simulink model "SYSTEMS"  (R2024b)
settings: configuration reference "STM32H7_Config" (kept outside this file)
settings Model: DataDictionary=Master_Dictionary.sldd  EnableAccessToBaseWorkspace=off  Creator=torni  LastModifiedBy=oxbro
settings ConfigSetRef: SourceName=STM32H7_Config

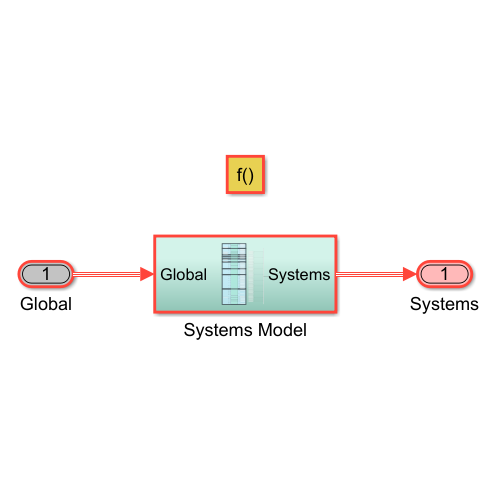
[thumbnail: Simulink's stored preview of the top-level diagram]
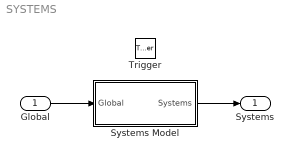
== system SYSTEMS ==
  "Global " : Inport  OutDataTypeStr=Bus: Global
  Trigger : TriggerPort  TriggerType=function-call  VariantControl=Variant  PortDimensions=1  TriggerSignalSampleTime=[0.003333333333333334,0]  OutDataTypeStr=double
  Systems Model : Subsystem
  Systems : Outport  OutDataTypeStr=Bus: SystemsBus  VectorParamsAs1DForOutWhenUnconnected=off
  wires:
  "Global "/1 -> Systems Model/1(Global)
  Systems Model/1(Systems) -> Systems/1

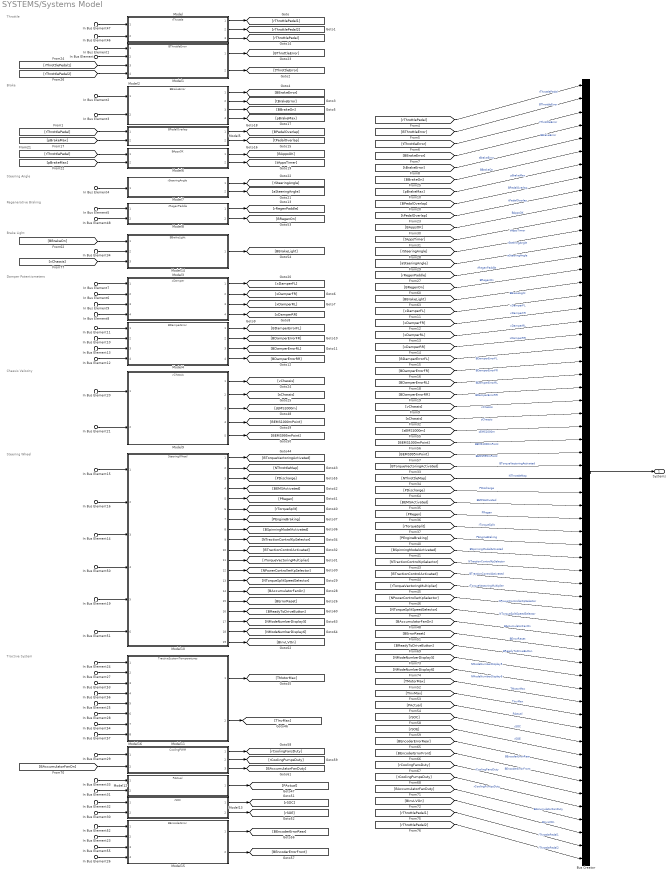
== system SYSTEMS/Systems Model ==
  note: Chassis Velocity
  note: Damper Potentiometers
  note: Regenerative Braking
  note: Steering Wheel
  note: Steering Angle
  note: Brake
  note: Throttle
  note: Tractive System
  note: Brake Light
  In Bus Element46 : Inport  PortName=Global  Element=SensorSignalsBus.VThrottlePedal2
  In Bus Element : Inport  PortName=Global  Element=SensorSignalsBus.VThrottlePedal2
  In Bus Element47 : Inport  PortName=Global  Element=SensorSignalsBus.VThrottlePedal1
  In Bus Element1 : Inport  PortName=Global  Element=SensorSignalsBus.VThrottlePedal1
  In Bus Element2 : Inport  PortName=Global  Element=SensorSignalsBus.pBrakeF
  In Bus Element3 : Inport  PortName=Global  Element=SensorSignalsBus.pBrakeR
  In Bus Element4 : Inport  PortName=Global  Element=SensorSignalsBus.VSteeringAngle
  In Bus Element5 : Inport  PortName=Global  Element=SensorSignalsBus.VRegenPaddle1
  In Bus Element48 : Inport  PortName=Global  Element=SensorSignalsBus.VRegenPaddle2
  In Bus Element6 : Inport  PortName=Global  Element=SensorSignalsBus.VDamperPotentiometerFR
  In Bus Element10 : Inport  PortName=Global  Element=SensorSignalsBus.VDamperPotentiometerFR
  In Bus Element7 : Inport  PortName=Global  Element=SensorSignalsBus.VDamperPotentiometerFL
  In Bus Element11 : Inport  PortName=Global  Element=SensorSignalsBus.VDamperPotentiometerFL
  In Bus Element8 : Inport  PortName=Global  Element=SensorSignalsBus.VDamperPotentiometerRR
  In Bus Element12 : Inport  PortName=Global  Element=SensorSignalsBus.VDamperPotentiometerRR
  In Bus Element9 : Inport  PortName=Global  Element=SensorSignalsBus.VDamperPotentiometerRL
  In Bus Element13 : Inport  PortName=Global  Element=SensorSignalsBus.VDamperPotentiometerRL
  In Bus Element16 : Inport  PortName=Global  Element=SensorSignalsBus.NDisplayNumberDDU7
  In Bus Element19 : Inport  PortName=Global  Element=SensorSignalsBus.BSteeringWheelButton4
  In Bus Element50 : Inport  PortName=Global  Element=SensorSignalsBus.BSteeringWheelButton5
  In Bus Element51 : Inport  PortName=Global  Element=SensorSignalsBus.BSteeringWheelButton6
  In Bus Element14 : Inport  PortName=Global  Element=SensorSignalsBus.BSteeringWheelButton2
  In Bus Element15 : Inport  PortName=Global  Element=SensorSignalsBus.BSteeringWheelButton7
  In Bus Element20 : Inport  PortName=Global  Element=WheelSpeedsBus.vWheelRL
  In Bus Element21 : Inport  PortName=Global  Element=WheelSpeedsBus.vWheelRR
  In Bus Element23 : Inport  PortName=Global  Element=InverterSignalsBus.InverterFLSignalsBus.NInvDTCFL
  In Bus Element24 : Inport  PortName=Global  Element=InverterSignalsBus.InverterFLSignalsBus.TMotorFL
  In Bus Element25 : Inport  PortName=Global  Element=InverterSignalsBus.InverterFLSignalsBus.TInvFL
  In Bus Element26 : Inport  PortName=Global  Element=InverterSignalsBus.InverterFRSignalsBus.NInvDTCFR
  In Bus Element27 : Inport  PortName=Global  Element=InverterSignalsBus.InverterFRSignalsBus.TMotorFR
  In Bus Element28 : Inport  PortName=Global  Element=InverterSignalsBus.InverterFRSignalsBus.TInvFR
  In Bus Element52 : Inport  PortName=Global  Element=InverterSignalsBus.InverterRLSignalsBus.NInvDTCRL
  In Bus Element53 : Inport  PortName=Global  Element=InverterSignalsBus.InverterRLSignalsBus.TMotorRL
  In Bus Element54 : Inport  PortName=Global  Element=InverterSignalsBus.InverterRLSignalsBus.TInvRL
  In Bus Element33 : Inport  PortName=Global  Element=InverterSignalsBus.InverterRLSignalsBus.VDCInvRL
  In Bus Element55 : Inport  PortName=Global  Element=InverterSignalsBus.InverterRRSignalsBus.NInvDTCRR
  In Bus Element56 : Inport  PortName=Global  Element=InverterSignalsBus.InverterRRSignalsBus.TMotorRR
  In Bus Element57 : Inport  PortName=Global  Element=InverterSignalsBus.InverterRRSignalsBus.TInvRR
  In Bus Element29 : Inport  PortName=Global  Element=BMSSignalsBus.TCellMax
  In Bus Element31 : Inport  PortName=Global  Element=BMSSignalsBus.IIVTS
  In Bus Element32 : Inport  PortName=Global  Element=BMSSignalsBus.IIVTS
  In Bus Element30 : Inport  PortName=Global  Element=BMSSignalsBus.VDCAccumulator
  In Bus Element34 : Inport  PortName=Global  Element=GPSIMUSignalsBus.gLongitudinalOXTSIMU
  Bus Creator : BusCreator  Inputs=60  OutDataTypeStr=Bus: SystemsBus
  Model : ModelReference  ModelNameDialog=rThrottle  SimulationMode=Normal  ModelReferenceVersion=13.5
  Model1 : ModelReference  ModelNameDialog=BThrottleError  SimulationMode=Normal  ModelReferenceVersion=13.5
  Model10 : ModelReference  ModelNameDialog=SteeringWheel.slx  SimulationMode=Normal  ModelReferenceVersion=13.5
  Model11 : ModelReference  ModelNameDialog=TractiveSystemTemperatures.slx  SimulationMode=Normal  ModelReferenceVersion=13.5
  Model12 : ModelReference  ModelNameDialog=PActual.slx  SimulationMode=Normal  ModelReferenceVersion=13.5
  Model13 : ModelReference  ModelNameDialog=rSOC.slx  SimulationMode=Normal  ModelReferenceVersion=13.5
  Model14 : ModelReference  ModelNameDialog=BBrakeLight.slx  SimulationMode=Normal  ModelReferenceVersion=13.5
  Model15 : ModelReference  ModelNameDialog=BEncoderError.slx  SimulationMode=Normal  ModelReferenceVersion=13.5
  Model16 : ModelReference  ModelNameDialog=CoolingPWM.slx  SimulationMode=Normal  ModelReferenceVersion=13.5
  Model2 : ModelReference  ModelNameDialog=BBrakeError  SimulationMode=Normal  ModelReferenceVersion=13.5
  Model3 : ModelReference  ModelNameDialog=xDamper  SimulationMode=Normal  ModelReferenceVersion=13.5
  Model4 : ModelReference  ModelNameDialog=BDamperError  SimulationMode=Normal  ModelReferenceVersion=13.5
  Model5 : ModelReference  ModelNameDialog=BPedalOverlap  SimulationMode=Normal  ModelReferenceVersion=13.5
  Model6 : ModelReference  ModelNameDialog=BAppsOK.slx  SimulationMode=Normal  ModelReferenceVersion=13.5
  Model7 : ModelReference  ModelNameDialog=rSteeringAngle.slx  SimulationMode=Normal  ModelReferenceVersion=13.5
  Model8 : ModelReference  ModelNameDialog=rRegenPaddle.slx  SimulationMode=Normal  ModelReferenceVersion=13.5
  Model9 : ModelReference  ModelNameDialog=vChassis.slx  SimulationMode=Normal  ModelReferenceVersion=13.5
  Systems : Outport  OutDataTypeStr=Bus: SystemsBus  VectorParamsAs1DForOutWhenUnconnected=off
  wires:
  In Bus Element47/1 -> Model/1
  In Bus Element46/1 -> Model/2
  In Bus Element/1 -> Model1/2
  In Bus Element1/1 -> Model1/1
  Model/1 -> [rThrottlePedal1]
  Model/2 -> [rThrottlePedal2]
  [rThrottlePedal1] -> Model1/3
  [rThrottlePedal2] -> Model1/4
  Model1/1 -> [BThrottleError]
  In Bus Element3/1 -> Model2/2
  In Bus Element2/1 -> Model2/1
  Model2/1 -> [BBrakeError]
  In Bus Element8/1 -> Model3/4
  In Bus Element9/1 -> Model3/3
  In Bus Element6/1 -> Model3/2
  In Bus Element7/1 -> Model3/1
  Model1/2 -> [tThrottleError]
  Model2/2 -> [tBrakeError]
  Model3/1 -> [xDamperFL]
  Model3/2 -> [xDamperFR]
  Model3/4 -> [xDamperRR]
  Model3/3 -> [xDamperRL]
  Model4/1 -> [BDamperErrorFL]
  Model4/2 -> [BDamperErrorFR]
  Model4/3 -> [BDamperErrorRL]
  Model4/4 -> [BDamperErrorRR]
  [rThrottlePedal] -> Model5/1
  Model5/2 -> [tPedalOverlap]
  Model5/1 -> [BPedalOverlap]
  [rThrottlePedal] -> Bus Creator/1  "rThrottlePedal"
  [BThrottleError] -> Bus Creator/2  "BThrottleError"
  [tThrottleError] -> Bus Creator/3  "tThrottleError"
  [BBrakeError] -> Bus Creator/4  "BBrakeError"
  [tBrakeError] -> Bus Creator/5  "tBrakeError"
  [xDamperFL] -> Bus Creator/17  "xDamperFL"
  [xDamperFR] -> Bus Creator/18  "xDamperFR"
  [xDamperRL] -> Bus Creator/19  "xDamperRL"
  [xDamperRR] -> Bus Creator/20  "xDamperRR"
  [BDamperErrorFL] -> Bus Creator/21  "BDamperErrorFL"
  [BDamperErrorFR] -> Bus Creator/22  "BDamperErrorFR"
  [BDamperErrorRL] -> Bus Creator/23  "BDamperErrorRL"
  [BDamperErrorRR] -> Bus Creator/24  "BDamperErrorRR"
  [BPedalOverlap] -> Bus Creator/8  "BPedalOverlap"
  [tPedalOverlap] -> Bus Creator/9  "tPedalOverlap"
  Bus Creator/1 -> Systems/1
  Model2/3 -> [BBrakeOn]
  [BBrakeOn] -> Bus Creator/6  "BBrakeOn"
  Model2/4 -> [pBrakeMax]
  [pBrakeMax] -> Model6/2
  [pBrakeMax] -> Model5/2
  Model6/1 -> [BAppsOK]
  Model6/2 -> [tAppsTimer]
  [rThrottlePedal] -> Model6/1
  Model/3 -> [rThrottlePedal]
  [rRegenPaddle] -> Bus Creator/14  "rRegenPaddle"
  Model8/1 -> [rRegenPaddle]
  Model7/1 -> [rSteeringAngle]
  Model7/2 -> [aSteeringAngle]
  [rSteeringAngle] -> Bus Creator/12  "rSteeringAngle"
  [aSteeringAngle] -> Bus Creator/13  "aSteeringAngle"
  In Bus Element21/1 -> Model9/2
  Model9/2 -> [sChassis]
  In Bus Element5/1 -> Model8/1
  In Bus Element48/1 -> Model8/2
  In Bus Element4/1 -> Model7/1
  In Bus Element19/1 -> Model10/5
  In Bus Element50/1 -> Model10/4
  In Bus Element51/1 -> Model10/6
  Model9/1 -> [vChassis]
  [vChassis] -> Bus Creator/25  "vChassis"
  [pBrakeMax] -> Bus Creator/7  "pBrakeMax"
  [BAppsOK] -> Bus Creator/10  "BAppsOK"
  [tAppsTimer] -> Bus Creator/11  "tAppsTimer"
  [sChassis] -> Bus Creator/26  "sChassis"
  [BTorqueVectoringActivated] -> Bus Creator/30  "BTorqueVectoringActivated"
  [NThrottleMap] -> Bus Creator/31  "NThrottleMap"
  [BEMSActivated] -> Bus Creator/33  "BEMSActivated"
  [PRegen] -> Bus Creator/34  "PRegen"
  [rTorqueSplit] -> Bus Creator/35  "rTorqueSplit"
  [PEngineBraking] -> Bus Creator/36  "PEngineBraking"
  [BSpinningModelActivated] -> Bus Creator/37  "BSpinningModelActivated"
  [NTractionControlKpSelector] -> Bus Creator/38  "NTractionControlKpSelector"
  [BTractionControlActivated] -> Bus Creator/39  "BTractionControlActivated"
  [rTorqueVectoringMultiplier] -> Bus Creator/40  "rTorqueVectoringMultiplier"
  [NPowerControllerKpSelector] -> Bus Creator/41  "NPowerControllerKpSelector"
  [NTorqueSplitSpeedSelector] -> Bus Creator/42  "NTorqueSplitSpeedSelector"
  [BAccumulatorFanOn] -> Bus Creator/43  "BAccumulatorFanOn"
  [BErrorReset] -> Bus Creator/44  "BErrorReset"
  In Bus Element24/1 -> Model11/1
  In Bus Element27/1 -> Model11/2
  In Bus Element53/1 -> Model11/3
  In Bus Element56/1 -> Model11/4
  In Bus Element28/1 -> Model11/6
  In Bus Element25/1 -> Model11/5
  In Bus Element54/1 -> Model11/7
  In Bus Element57/1 -> Model11/8
  [TMotorMax] -> Bus Creator/48  "TMotorMax"
  [TInvMax] -> Bus Creator/49  "TInvMax"
  In Bus Element33/1 -> Model12/1
  In Bus Element31/1 -> Model12/2
  Model12/1 -> [PActual]
  [PActual] -> Bus Creator/50  "PActual"
  Model9/3 -> [sEMS1000m]
  Model9/4 -> [BEMS1000mPoint]
  Model9/5 -> [BEMS995mPoint]
  [sEMS1000m] -> Bus Creator/27  "sEMS1000m"
  [BEMS1000mPoint] -> Bus Creator/28  "BEMS1000mPoint"
  [BEMS995mPoint] -> Bus Creator/29  "BEMS995mPoint"
  In Bus Element32/1 -> Model13/1
  In Bus Element30/1 -> Model13/2
  Model13/1 -> [rSOC]
  Model13/2 -> [rSOE]
  [rSOC] -> Bus Creator/51  "rSOC"
  [rSOE] -> Bus Creator/52  "rSOE"
  Model8/2 -> [BRegenOn]
  [BRegenOn] -> Bus Creator/15  "BRegenOn"
  [BBrakeOn] -> Model14/1
  Model14/1 -> [BBrakeLight]
  [BBrakeLight] -> Bus Creator/16  "BBrakeLight"
  [PDischarge] -> Bus Creator/32  "PDischarge"
  In Bus Element52/1 -> Model15/1
  In Bus Element55/1 -> Model15/3
  In Bus Element26/1 -> Model15/4
  In Bus Element23/1 -> Model15/2
  Model15/1 -> [BEncoderErrorRear]
  Model15/2 -> [BEncoderErrorFront]
  [BEncoderErrorRear] -> Bus Creator/53  "BEncoderErrorRear"
  [BEncoderErrorFront] -> Bus Creator/54  "BEncoderErrorFront"
  Model16/1 -> [rCoolingFansDuty]
  Model16/2 -> [rCoolingPumpsDuty]
  [rCoolingFansDuty] -> Bus Creator/55  "rCoolingFansDuty"
  [rCoolingPumpsDuty] -> Bus Creator/56  "rCoolingPumpsDuty"
  [BReadyToDriveButton] -> Bus Creator/45  "BReadyToDriveButton"
  Model16/3 -> [BAccumulatorFanDuty]
  In Bus Element29/1 -> Model16/1
  [BAccumulatorFanOn] -> Model16/2
  [BAccumulatorFanDuty] -> Bus Creator/57  "BAccumulatorFanDuty"
  [NModeNumberDisplay5] -> Bus Creator/46  "NModeNumberDisplay5"
  [NModeNumberDisplay6] -> Bus Creator/47  "NModeNumberDisplay6"
  In Bus Element11/1 -> Model4/1
  In Bus Element10/1 -> Model4/2
  In Bus Element13/1 -> Model4/3
  In Bus Element12/1 -> Model4/4
  In Bus Element16/1 -> Model10/2
  Model10/1 -> [BTorqueVectoringActivated]
  Model10/2 -> [NThrottleMap]
  Model10/3 -> [PDischarge]
  Model10/4 -> [BEMSActivated]
  Model10/5 -> [PRegen]
  Model10/6 -> [rTorqueSplit]
  Model10/7 -> [PEngineBraking]
  Model10/8 -> [BSpinningModelActivated]
  Model10/9 -> [NTractionControlKpSelector]
  Model10/10 -> [BTractionControlActivated]
  Model10/11 -> [rTorqueVectoringMultiplier]
  Model10/12 -> [NPowerControllerKpSelector]
  Model10/13 -> [NTorqueSplitSpeedSelector]
  Model10/14 -> [BAccumulatorFanOn]
  Model10/15 -> [BErrorReset]
  Model10/16 -> [BReadyToDriveButton]
  Model10/17 -> [NModeNumberDisplay5]
  Model10/18 -> [NModeNumberDisplay6]
  In Bus Element34/1 -> Model14/2
  Model10/19 -> [BInvLVOn]
  [BInvLVOn] -> Bus Creator/58  "BInvLVOn"
  [rThrottlePedal1] -> Bus Creator/59  "rThrottlePedal1"
  [rThrottlePedal2] -> Bus Creator/60  "rThrottlePedal2"
  [vChassis] -> Model14/3
  Model11/2 -> [TInvMax]
  Model11/1 -> [TMotorMax]
  In Bus Element20/1 -> Model9/1
  In Bus Element14/1 -> Model10/3
  In Bus Element15/1 -> Model10/1
